simulink model "UART_test"  (R2020a)
settings: Solver=FixedStepAuto  StartTime=0.0  StopTime=10.0  FixedStep=1e-3  RelTol=1e-3  EnableMultiTasking=on
libraries: etargetslib x17, frdmk64flib x10, simulink x1
(part 2 of 3)

== stateflow chart UART_test/Pacing Modes ==
  state Pacing_Off
    % do nothing
  state Pacing_Modes_Switch
    % switch pacing modes according to MODE
    % This is similar to switch case structure in C plus plus
    % this block is executed only after mode is switched or pparams are updated
    entry:
    % Reset LEDs
    R_LED=false;
    G_LED=false;
    B_LED=false;
    % reset output variables before switching mode
    VENT_CMP_REF_PWM=100;
    ATR_CMP_REF_PWM=100;
    FRONTEND_CTRL=true;
    ATR_PACE_CTRL = false;
    VENT_PACE_CTRL = false;
    PACING_REF_PWM = 0;
    PACE_CHARGE_CTRL = false;
    PACE_GND_CTRL = false;
    Z_ATR_CTRL = false;
    Z_VENT_CTRL = false;
    ATR_GND_CTRL = false;
    VENT_GND_CTRL = false;
    % Update internal double representations of input parameters
    % Note: MODE and ACT_THRESHOLD don't need to be double
    % MODE=double(MODE_i);
    LRL=double(LRL_i);
    URL=double(URL_i);
    MAX_SENSOR_RATE=double(MAX_SENSOR_RATE_i);
    AV_DELAY_FIXED=double(AV_DELAY_FIXED_i);
    AV_DELAY_DYNAMIC=double(AV_DELAY_DYNAMIC_i);
    MIN_AV_DELAY_DYNAMIC=double(MIN_AV_DELAY_DYNAMIC_i);
    AV_DELAY_OFFSET_SENSED=double(AV_DELAY_OFFSET_SENSED_i);
    ATR_AMP_REG=double(ATR_AMP_REG_i);
    VENT_AMP_REG=double(VENT_AMP_REG_i);
    ATR_AMP_UNREG=double(ATR_AMP_UNREG_i);
    VENT_AMP_UNREG=double(VENT_AMP_UNREG_i);
    ATR_PULSE_WIDTH=double(ATR_PULSE_WIDTH_i);
    VENT_PULSE_WIDTH=double(VENT_PULSE_WIDTH_i);
    ATR_SENSITIVITY=double(ATR_SENSITIVITY_i);
    VENT_SENSITIVITY=double(VENT_SENSITIVITY_i);
    VRP=double(VRP_i);
    ARP=double(ARP_i);
    PVARP=double(PVARP_i);
    PVARP_EXT=double(PVARP_EXT_i);
    HYSTERESIS_LIMIT=double(HYSTERESIS_LIMIT_i);
    RATE_SMOOTHING=double(RATE_SMOOTHING_i);
    ATR_MODE=double(ATR_MODE_i);
    ATR_DURATION=double(ATR_DURATION_i);
    ATR_FALLBACK_TIME=double(ATR_FALLBACK_TIME_i);
    VENT_BLANKING=double(VENT_BLANKING_i);
    % ACT_THRESHOLD=double(ACT_THRESHOLD_i);
    REACTION_TIME=double(REACTION_TIME_i);
    RESPONSE_FACTOR=double(RESPONSE_FACTOR_i);
    RECOVERY_TIME=double(RECOVERY_TIME_i);
  state DOO
    note: DOO Pacing Mode:
        | equivalent to AOO combined with VOO, but with a AV_Delay
    state Atrium_Pacing
      entry:
      % VENT_PACE_CTRL = false;
      % ATR_GND_CTRL = false;
      VENT_GND_CTRL = false;
      PACE_CHARGE_CTRL = false;
      % starting pacing at last step to be secure
      ATR_PACE_CTRL = true;
    state Atrium_Charging
      %% Charge C22
      entry:
      % ATR_PACE_CTRL = false;
      VENT_PACE_CTRL = false;
      ATR_GND_CTRL = false;
      %% discharge residual voltage inside ventricle
      VENT_GND_CTRL = true;
      % Because 0-100% PWM corresponds to 0-5V output,
      % PWM duty cycle = ATR_AMP_REG/5*100;
      PACING_REF_PWM = ATR_AMP_REG*20;
      PACE_CHARGE_CTRL = true;
    state Init
      % Initialize
      entry:
      %% C21 is always connected
      PACE_GND_CTRL = true;
      Z_ATR_CTRL = false;
      Z_VENT_CTRL = false;
    state Ventricle_Pacing
      entry:
      % ATR_PACE_CTRL = false;
      ATR_GND_CTRL = false;
      % VENT_GND_CTRL = false;
      PACE_CHARGE_CTRL = false;
      % starting pacing at last step to be secure
      VENT_PACE_CTRL = true;
    state Ventricle_Charging
      % charge C22
      entry:
      ATR_PACE_CTRL = false;
      % VENT_PACE_CTRL = false;
      %% discharge residual voltage inside atrium
      ATR_GND_CTRL = true;
      VENT_GND_CTRL = false;
      % Because 0-100% PWM corresponds to 0-5V output,
      %PWM duty cycle = VENT_AMP_REG/5*100;
      PACING_REF_PWM = VENT_AMP_REG*20;
      PACE_CHARGE_CTRL = true;
    (default) -> DOO.Init
    DOO.Atrium_Charging -> DOO.Atrium_Pacing : [after(60000/LRL-ATR_PULSE_WIDTH-AV_DELAY_FIXED-VENT_PULSE_WIDTH,msec)]
    DOO.Init -> DOO.Atrium_Charging
    DOO.Atrium_Pacing -> DOO.Ventricle_Charging : [after(ATR_PULSE_WIDTH,msec)]
    DOO.Ventricle_Pacing -> DOO.Atrium_Charging : [after(VENT_PULSE_WIDTH,msec)]
    DOO.Ventricle_Charging -> DOO.Ventricle_Pacing : [after(AV_DELAY_FIXED,msec)]
  state AOO
    note: AOO Pacing Mode:
        |
        | Inputs:
        | ppm=LRL; (1/automatic interval)
        | ATR_AMP_REG; (amplitude in V)
        | ATR_PULSE_WIDTH; (in msec)
    state Charging
      %% Charge C22
      entry:
      ATR_PACE_CTRL = false;
      ATR_GND_CTRL = true;
      % Because 0-100% PWM corresponds to 0-5V output,
      % PWM duty cycle = ATR_AMP_REG/5*100;
      PACING_REF_PWM = ATR_AMP_REG*20;
      PACE_CHARGE_CTRL = true;
    state Pacing
      entry:
      ATR_GND_CTRL = false;
      PACE_CHARGE_CTRL = false;
      % start pacing at last step to be secure
      ATR_PACE_CTRL = true;
    state Init
      % Initialize
      entry:
      %% C21 is always connected
      PACE_GND_CTRL = true;
      Z_ATR_CTRL = false;
      Z_VENT_CTRL = false;
      VENT_GND_CTRL = false;
      VENT_PACE_CTRL = false;
    (default) -> AOO.Init
    AOO.Charging -> AOO.Pacing : [after(60000/LRL-ATR_PULSE_WIDTH,msec)]
    AOO.Init -> AOO.Charging
    AOO.Pacing -> AOO.Charging : [after(ATR_PULSE_WIDTH,msec)]
  state DOOR
    state Very_High_Threshold
      entry:
      % assign predefined constant
      ACT_THRESHOLD=ACT_V_HIGH;
    state High_Threshold
      entry:
      ACT_THRESHOLD=ACT_HIGH;
    state Init
      entry:
      % initialize constants that will be used in the ..._Cycle
      BPM = LRL;
      % MSR_ALTERED: max sensor rate altered to be smaller than either limit (MSR or URL)
      MSR_ALTERED=min(MAX_SENSOR_RATE,URL);
      % difference between MSR and LRL
      DIFF_MSR_LRL=MSR_ALTERED-LRL;
      % target and slope for BPM when activity higher/lower than threshold
      TARGET_HIGH = DIFF_MSR_LRL * (RESPONSE_FACTOR/16) + LRL;
      TARGET_LOW = LRL;
      SLOPE_UP=DIFF_MSR_LRL/REACTION_TIME;
      SLOPE_DOWN=DIFF_MSR_LRL/RECOVERY_TIME;
      % Note: both reaction and recovery time are in seconds
    state Medium_High_Threshold
      entry:
      ACT_THRESHOLD=ACT_M_HIGH;
    state DOOR_Cycle
      state BPM_Update [parallel]
        settings: executionOrder=1
        state Get_activity
          entry:
          ACTIVITY_NORM = sqrt(ACTIVITY(1)^2+ACTIVITY(2)^2+ACTIVITY(3)^2);
        state More_than_threshold
        state Less_than_threshold
        state Increse_HR
          entry:
          % step is change in BPM after every pace
          % the last step should be smaller to let BPM reach TARGET exactly
          STEP=min(SLOPE_UP*(60/BPM),TARGET_HIGH-BPM);
          BPM = BPM + STEP;
          B_LED=true;
          R_LED=false;
          G_LED=false;
        state Decrese_HR
          entry:
          % step is change in BPM after every pace
          % the last step should be smaller to let BPM reach TARGET exactly
          STEP=min(SLOPE_DOWN*(60/BPM),BPM-TARGET_LOW);
          BPM = BPM - STEP;
          G_LED=true;
          R_LED=false;
          B_LED=false;
        state Maintain_HR
          % no change to BPM
          entry:
          R_LED=true;
          G_LED=false;
          B_LED=false;
        (default) -> DOOR.DOOR_Cycle.BPM_Update.Get_activity
        (junction 1173) -> DOOR.DOOR_Cycle.BPM_Update.Get_activity : [after(60/BPM,sec)]
        DOOR.DOOR_Cycle.BPM_Update.Get_activity -> DOOR.DOOR_Cycle.BPM_Update.More_than_threshold [order 2] : [ACTIVITY_NORM >= ACT_THRESHOLD]
        DOOR.DOOR_Cycle.BPM_Update.Get_activity -> DOOR.DOOR_Cycle.BPM_Update.Less_than_threshold [order 1] : [ACTIVITY_NORM< ACT_THRESHOLD]
        DOOR.DOOR_Cycle.BPM_Update.Less_than_threshold -> DOOR.DOOR_Cycle.BPM_Update.Maintain_HR [order 2]
        DOOR.DOOR_Cycle.BPM_Update.Less_than_threshold -> DOOR.DOOR_Cycle.BPM_Update.Decrese_HR [order 1] : [BPM > TARGET_LOW]
        DOOR.DOOR_Cycle.BPM_Update.More_than_threshold -> DOOR.DOOR_Cycle.BPM_Update.Increse_HR [order 1] : [BPM < TARGET_HIGH]
        DOOR.DOOR_Cycle.BPM_Update.More_than_threshold -> DOOR.DOOR_Cycle.BPM_Update.Maintain_HR [order 2]
        DOOR.DOOR_Cycle.BPM_Update.Increse_HR -> (junction 1173)
        DOOR.DOOR_Cycle.BPM_Update.Maintain_HR -> (junction 1173)
        DOOR.DOOR_Cycle.BPM_Update.Decrese_HR -> (junction 1173)
      state DOO_Timing_Logic [parallel]
        settings: executionOrder=2
        note: DOO Pacing Mode:
            | equivalent to AOO combined with VOO, but with a AV_Delay
        state Atrium_Pacing
          entry:
          % VENT_PACE_CTRL = false;
          % ATR_GND_CTRL = false;
          VENT_GND_CTRL = false;
          PACE_CHARGE_CTRL = false;
          % starting pacing at last step to be secure
          ATR_PACE_CTRL = true;
        state Atrium_Charging
          %% Charge C22
          entry:
          % ATR_PACE_CTRL = false;
          VENT_PACE_CTRL = false;
          ATR_GND_CTRL = false;
          %% discharge residual voltage inside ventricle
          VENT_GND_CTRL = true;
          % Because 0-100% PWM corresponds to 0-5V output,
          % PWM duty cycle = ATR_AMP_REG/5*100;
          PACING_REF_PWM = ATR_AMP_REG*20;
          PACE_CHARGE_CTRL = true;
        state Init
          % Initialize
          entry:
          %% C21 is always connected
          PACE_GND_CTRL = true;
          Z_ATR_CTRL = false;
          Z_VENT_CTRL = false;
        state Ventricle_Pacing
          entry:
          % ATR_PACE_CTRL = false;
          ATR_GND_CTRL = false;
          % VENT_GND_CTRL = false;
          PACE_CHARGE_CTRL = false;
          % starting pacing at last step to be secure
          VENT_PACE_CTRL = true;
        state Ventricle_Charging
          % charge C22
          entry:
          ATR_PACE_CTRL = false;
          % VENT_PACE_CTRL = false;
          %% discharge residual voltage inside atrium
          ATR_GND_CTRL = true;
          VENT_GND_CTRL = false;
          % Because 0-100% PWM corresponds to 0-5V output,
          %PWM duty cycle = VENT_AMP_REG/5*100;
          PACING_REF_PWM = VENT_AMP_REG*20;
          PACE_CHARGE_CTRL = true;
        (default) -> DOOR.DOOR_Cycle.DOO_Timing_Logic.Init
        DOOR.DOOR_Cycle.DOO_Timing_Logic.Atrium_Charging -> DOOR.DOOR_Cycle.DOO_Timing_Logic.Atrium_Pacing : [after(60000/BPM - ATR_PULSE_WIDTH - AV_DELAY_FIXED - VENT_PULSE_WIDTH,msec)]
        DOOR.DOOR_Cycle.DOO_Timing_Logic.Init -> DOOR.DOOR_Cycle.DOO_Timing_Logic.Atrium_Charging
        DOOR.DOOR_Cycle.DOO_Timing_Logic.Atrium_Pacing -> DOOR.DOOR_Cycle.DOO_Timing_Logic.Ventricle_Charging : [after(ATR_PULSE_WIDTH,msec)]
        DOOR.DOOR_Cycle.DOO_Timing_Logic.Ventricle_Pacing -> DOOR.DOOR_Cycle.DOO_Timing_Logic.Atrium_Charging : [after(VENT_PULSE_WIDTH,msec)]
        DOOR.DOOR_Cycle.DOO_Timing_Logic.Ventricle_Charging -> DOOR.DOOR_Cycle.DOO_Timing_Logic.Ventricle_Pacing : [after(AV_DELAY_FIXED,msec)]
    state Medium_Threshold
      % if no match value for ACT_THRESHOLD, use medium as default
      entry:
      ACT_THRESHOLD=ACT_M;
    state Medium_Low_Threshold
      entry:
      ACT_THRESHOLD=ACT_M_LOW;
    state Low_Threshold
      entry:
      ACT_THRESHOLD=ACT_LOW;
    state Very_Low_Threshold
      entry:
      ACT_THRESHOLD=ACT_V_LOW;
    (default) -> DOOR.Init
    DOOR.Very_High_Threshold -> DOOR_Cycle
    (junction 1150) -> DOOR.Very_High_Threshold [order 1] : [ACT_THRESHOLD_i==6]
    (junction 1150) -> DOOR.High_Threshold [order 2] : [ACT_THRESHOLD_i==5]
    DOOR.High_Threshold -> DOOR_Cycle
    DOOR.Medium_High_Threshold -> DOOR_Cycle
    (junction 1150) -> DOOR.Medium_High_Threshold [order 5] : [ACT_THRESHOLD_i==4]
    DOOR.Init -> (junction 1150)
    (junction 1150) -> DOOR.Medium_Threshold [order 7]
    DOOR.Medium_Threshold -> DOOR_Cycle
    (junction 1150) -> DOOR.Medium_Low_Threshold [order 4] : [ACT_THRESHOLD_i==2]
    (junction 1150) -> DOOR.Low_Threshold [order 3] : [ACT_THRESHOLD_i==1]
    (junction 1150) -> DOOR.Very_Low_Threshold [order 6] : [ACT_THRESHOLD_i==0]
    DOOR.Low_Threshold -> DOOR_Cycle
    DOOR.Medium_Low_Threshold -> DOOR_Cycle
    DOOR.Very_Low_Threshold -> DOOR_Cycle
  state AOOR
    state Very_High_Threshold
      entry:
      % assign predefined constant
      ACT_THRESHOLD=ACT_V_HIGH;
    state High_Threshold
      entry:
      ACT_THRESHOLD=ACT_HIGH;
    state Init
      entry:
      % initialize constants that will be used in the ..._Cycle
      BPM = LRL;
      % MSR_ALTERED: max sensor rate altered to be smaller than either limit (MSR or URL)
      MSR_ALTERED=min(MAX_SENSOR_RATE,URL);
      % difference between MSR and LRL
      DIFF_MSR_LRL=MSR_ALTERED-LRL;
      % target and slope for BPM when activity higher/lower than threshold
      TARGET_HIGH = DIFF_MSR_LRL * (RESPONSE_FACTOR/16) + LRL;
      TARGET_LOW = LRL;
      SLOPE_UP=DIFF_MSR_LRL/REACTION_TIME;
      SLOPE_DOWN=DIFF_MSR_LRL/RECOVERY_TIME;
      % Note: both reaction and recovery time are in seconds
    state Medium_High_Threshold
      entry:
      ACT_THRESHOLD=ACT_M_HIGH;
    state AOOR_Cycle
      state BPM_Update [parallel]
        settings: executionOrder=1
        state Get_activity
          entry:
          ACTIVITY_NORM = sqrt(ACTIVITY(1)^2+ACTIVITY(2)^2+ACTIVITY(3)^2);
        state More_than_threshold
        state Less_than_threshold
        state Increse_HR
          entry:
          % step is change in BPM after every pace
          % the last step should be smaller to let BPM reach TARGET exactly
          STEP=min(SLOPE_UP*(60/BPM),TARGET_HIGH-BPM);
          BPM = BPM + STEP;
          B_LED=true;
          R_LED=false;
          G_LED=false;
        state Decrese_HR
          entry:
          % step is change in BPM after every pace
          % the last step should be smaller to let BPM reach TARGET exactly
          STEP=min(SLOPE_DOWN*(60/BPM),BPM-TARGET_LOW);
          BPM = BPM - STEP;
          G_LED=true;
          R_LED=false;
          B_LED=false;
        state Maintain_HR
          % no change to BPM
          entry:
          R_LED=true;
          G_LED=false;
          B_LED=false;
        (default) -> AOOR.AOOR_Cycle.BPM_Update.Get_activity
        (junction 803) -> AOOR.AOOR_Cycle.BPM_Update.Get_activity : [after(60/BPM,sec)]
        AOOR.AOOR_Cycle.BPM_Update.Get_activity -> AOOR.AOOR_Cycle.BPM_Update.More_than_threshold [order 2] : [ACTIVITY_NORM >= ACT_THRESHOLD]
        AOOR.AOOR_Cycle.BPM_Update.Get_activity -> AOOR.AOOR_Cycle.BPM_Update.Less_than_threshold [order 1] : [ACTIVITY_NORM< ACT_THRESHOLD]
        AOOR.AOOR_Cycle.BPM_Update.Less_than_threshold -> AOOR.AOOR_Cycle.BPM_Update.Maintain_HR [order 2]
        AOOR.AOOR_Cycle.BPM_Update.Less_than_threshold -> AOOR.AOOR_Cycle.BPM_Update.Decrese_HR [order 1] : [BPM > TARGET_LOW]
        AOOR.AOOR_Cycle.BPM_Update.More_than_threshold -> AOOR.AOOR_Cycle.BPM_Update.Increse_HR [order 1] : [BPM < TARGET_HIGH]
        AOOR.AOOR_Cycle.BPM_Update.More_than_threshold -> AOOR.AOOR_Cycle.BPM_Update.Maintain_HR [order 2]
        AOOR.AOOR_Cycle.BPM_Update.Increse_HR -> (junction 803)
        AOOR.AOOR_Cycle.BPM_Update.Maintain_HR -> (junction 803)
        AOOR.AOOR_Cycle.BPM_Update.Decrese_HR -> (junction 803)
      state AOO_Timing_Logic [parallel]
        settings: executionOrder=2
        note: AOO Pacing Mode:
            |
            | Inputs:
            | ppm=LRL; (1/automatic interval)
            | ATR_AMP_REG; (amplitude in V)
            | ATR_PULSE_WIDTH; (in msec)
        state Charging
          %% Charge C22
          entry:
          ATR_PACE_CTRL = false;
          ATR_GND_CTRL = true;
          % Because 0-100% PWM corresponds to 0-5V output,
          % PWM duty cycle = ATR_AMP_REG/5*100;
          PACING_REF_PWM = ATR_AMP_REG*20;
          PACE_CHARGE_CTRL = true;
        state Pacing
          entry:
          ATR_GND_CTRL = false;
          PACE_CHARGE_CTRL = false;
          ATR_PACE_CTRL = true;
        state Init
          % Initialize
          entry:
          %% C21 is always connected
          PACE_GND_CTRL = true;
          Z_ATR_CTRL = false;
          Z_VENT_CTRL = false;
          VENT_GND_CTRL = false;
          VENT_PACE_CTRL = false;
        (default) -> AOOR.AOOR_Cycle.AOO_Timing_Logic.Init
        AOOR.AOOR_Cycle.AOO_Timing_Logic.Charging -> AOOR.AOOR_Cycle.AOO_Timing_Logic.Pacing : [after(60000/BPM-ATR_PULSE_WIDTH,msec)]
        AOOR.AOOR_Cycle.AOO_Timing_Logic.Init -> AOOR.AOOR_Cycle.AOO_Timing_Logic.Charging
        AOOR.AOOR_Cycle.AOO_Timing_Logic.Pacing -> AOOR.AOOR_Cycle.AOO_Timing_Logic.Charging : [after(ATR_PULSE_WIDTH,msec)]
    state Medium_Threshold
      % if no match value for ACT_THRESHOLD, use medium as default
      entry:
      ACT_THRESHOLD=ACT_M;
    state Medium_Low_Threshold
      entry:
      ACT_THRESHOLD=ACT_M_LOW;
    state Low_Threshold
      entry:
      ACT_THRESHOLD=ACT_LOW;
    state Very_Low_Threshold
      entry:
      ACT_THRESHOLD=ACT_V_LOW;
    (default) -> AOOR.Init
    AOOR.Very_High_Threshold -> AOOR_Cycle
    (junction 148) -> AOOR.Very_High_Threshold [order 1] : [ACT_THRESHOLD_i==6]
    (junction 148) -> AOOR.High_Threshold [order 2] : [ACT_THRESHOLD_i==5]
    AOOR.High_Threshold -> AOOR_Cycle
    AOOR.Medium_High_Threshold -> AOOR_Cycle
    (junction 148) -> AOOR.Medium_High_Threshold [order 5] : [ACT_THRESHOLD_i==4]
    AOOR.Init -> (junction 148)
    (junction 148) -> AOOR.Medium_Threshold [order 7]
    AOOR.Medium_Threshold -> AOOR_Cycle
    (junction 148) -> AOOR.Medium_Low_Threshold [order 4] : [ACT_THRESHOLD_i==2]
    (junction 148) -> AOOR.Low_Threshold [order 3] : [ACT_THRESHOLD_i==1]
    (junction 148) -> AOOR.Very_Low_Threshold [order 6] : [ACT_THRESHOLD_i==0]
    AOOR.Low_Threshold -> AOOR_Cycle
    AOOR.Medium_Low_Threshold -> AOOR_Cycle
    AOOR.Very_Low_Threshold -> AOOR_Cycle
  state VOO
    note: VOO Pacing Mode:
        |
        | Inputs:
        | ppm=LRL; (1/automatic interval)
        | VENT_AMP_REG; (amplitude in V)
        | VENT_PULSE_WIDTH; (in msec)
    state Charging1
      %% Charge C22
      entry:
      VENT_PACE_CTRL = false;
      VENT_GND_CTRL = true;
      % Because 0-100% PWM corresponds to 0-5V output,
      % PWM duty cycle = VENT_AMP_REG/5*100;
      PACING_REF_PWM = VENT_AMP_REG*20;
      PACE_CHARGE_CTRL = true;
    state Pacing1
      entry:
      VENT_GND_CTRL = false;
      PACE_CHARGE_CTRL = false;
      % start pacing at last step to be secure
      VENT_PACE_CTRL = true;
    state Init
      % Initialize
      entry:
      %% C21 is always connected
      PACE_GND_CTRL = true;
      Z_ATR_CTRL = false;
      Z_VENT_CTRL = false;
      ATR_GND_CTRL = false;
      ATR_PACE_CTRL = false;
    (default) -> VOO.Init
    VOO.Charging1 -> VOO.Pacing1 : [after(60000/LRL-VENT_PULSE_WIDTH,msec)]
    VOO.Init -> VOO.Charging1
    VOO.Pacing1 -> VOO.Charging1 : [after(VENT_PULSE_WIDTH,msec)]
  state VOOR
    state Very_High_Threshold
      entry:
      % assign predefined constant
      ACT_THRESHOLD=ACT_V_HIGH;
    state High_Threshold
      entry:
      ACT_THRESHOLD=ACT_HIGH;
    state Init
      entry:
      % initialize constants that will be used in the ..._Cycle
      BPM = LRL;
      % MSR_ALTERED: max sensor rate altered to be smaller than either limit (MSR or URL)
      MSR_ALTERED=min(MAX_SENSOR_RATE,URL);
      % difference between MSR and LRL
      DIFF_MSR_LRL=MSR_ALTERED-LRL;
      % target and slope for BPM when activity higher/lower than threshold
      TARGET_HIGH = DIFF_MSR_LRL * (RESPONSE_FACTOR/16) + LRL;
      TARGET_LOW = LRL;
      SLOPE_UP=DIFF_MSR_LRL/REACTION_TIME;
      SLOPE_DOWN=DIFF_MSR_LRL/RECOVERY_TIME;
      % Note: both reaction and recovery time are in seconds
    state Medium_High_Threshold
      entry:
      ACT_THRESHOLD=ACT_M_HIGH;
    state VOOR_Cycle
      state BPM_Update [parallel]
        settings: executionOrder=1
        state Get_activity
          entry:
          ACTIVITY_NORM = sqrt(ACTIVITY(1)^2+ACTIVITY(2)^2+ACTIVITY(3)^2);
        state More_than_threshold
        state Less_than_threshold
        state Increse_HR
          entry:
          % step is change in BPM after every pace
          % the last step should be smaller to let BPM reach TARGET exactly
          STEP=min(SLOPE_UP*(60/BPM),TARGET_HIGH-BPM);
          BPM = BPM + STEP;
          B_LED=true;
          R_LED=false;
          G_LED=false;
        state Decrese_HR
          entry:
          % step is change in BPM after every pace
          % the last step should be smaller to let BPM reach TARGET exactly
          STEP=min(SLOPE_DOWN*(60/BPM),BPM-TARGET_LOW);
          BPM = BPM - STEP;
          G_LED=true;
          R_LED=false;
          B_LED=false;
        state Maintain_HR
          % no change to BPM
          entry:
          R_LED=true;
          G_LED=false;
          B_LED=false;
        (default) -> VOOR.VOOR_Cycle.BPM_Update.Get_activity
        (junction 972) -> VOOR.VOOR_Cycle.BPM_Update.Get_activity : [after(60/BPM,sec)]
        VOOR.VOOR_Cycle.BPM_Update.Get_activity -> VOOR.VOOR_Cycle.BPM_Update.More_than_threshold [order 2] : [ACTIVITY_NORM >= ACT_THRESHOLD]
        VOOR.VOOR_Cycle.BPM_Update.Get_activity -> VOOR.VOOR_Cycle.BPM_Update.Less_than_threshold [order 1] : [ACTIVITY_NORM< ACT_THRESHOLD]
        VOOR.VOOR_Cycle.BPM_Update.Less_than_threshold -> VOOR.VOOR_Cycle.BPM_Update.Maintain_HR [order 2]
        VOOR.VOOR_Cycle.BPM_Update.Less_than_threshold -> VOOR.VOOR_Cycle.BPM_Update.Decrese_HR [order 1] : [BPM > TARGET_LOW]
        VOOR.VOOR_Cycle.BPM_Update.More_than_threshold -> VOOR.VOOR_Cycle.BPM_Update.Increse_HR [order 1] : [BPM < TARGET_HIGH]
        VOOR.VOOR_Cycle.BPM_Update.More_than_threshold -> VOOR.VOOR_Cycle.BPM_Update.Maintain_HR [order 2]
        VOOR.VOOR_Cycle.BPM_Update.Increse_HR -> (junction 972)
        VOOR.VOOR_Cycle.BPM_Update.Maintain_HR -> (junction 972)
        VOOR.VOOR_Cycle.BPM_Update.Decrese_HR -> (junction 972)
      state VOO_Timing_Logic [parallel]
        settings: executionOrder=2
        note: VOO Pacing Mode:
            |
            | Inputs:
            | ppm=LRL; (1/automatic interval)
            | VENT_AMP_REG; (amplitude in V)
            | VENT_PULSE_WIDTH; (in msec)
        state Charging1
          %% Charge C22
          entry:
          VENT_PACE_CTRL = false;
          VENT_GND_CTRL = true;
          % Because 0-100% PWM corresponds to 0-5V output,
          % PWM duty cycle = VENT_AMP_REG/5*100;
          PACING_REF_PWM = VENT_AMP_REG*20;
          PACE_CHARGE_CTRL = true;
        state Pacing1
          entry:
          VENT_GND_CTRL = false;
          PACE_CHARGE_CTRL = false;
          % start pacing at last step to be secure
          VENT_PACE_CTRL = true;
        state Init
          % Initialize
          entry:
          %% C21 is always connected
          PACE_GND_CTRL = true;
          Z_ATR_CTRL = false;
          Z_VENT_CTRL = false;
          ATR_GND_CTRL = false;
          ATR_PACE_CTRL = false;
        (default) -> VOOR.VOOR_Cycle.VOO_Timing_Logic.Init
        VOOR.VOOR_Cycle.VOO_Timing_Logic.Charging1 -> VOOR.VOOR_Cycle.VOO_Timing_Logic.Pacing1 : [after(60000/BPM-VENT_PULSE_WIDTH,msec)]
        VOOR.VOOR_Cycle.VOO_Timing_Logic.Init -> VOOR.VOOR_Cycle.VOO_Timing_Logic.Charging1
        VOOR.VOOR_Cycle.VOO_Timing_Logic.Pacing1 -> VOOR.VOOR_Cycle.VOO_Timing_Logic.Charging1 : [after(VENT_PULSE_WIDTH,msec)]
    state Medium_Threshold
      % if no match value for ACT_THRESHOLD, use medium as default
      entry:
      ACT_THRESHOLD=ACT_M;
    state Medium_Low_Threshold
      entry:
      ACT_THRESHOLD=ACT_M_LOW;
    state Low_Threshold
      entry:
      ACT_THRESHOLD=ACT_LOW;
    state Very_Low_Threshold
      entry:
      ACT_THRESHOLD=ACT_V_LOW;
    (default) -> VOOR.Init
    VOOR.Very_High_Threshold -> VOOR_Cycle
    (junction 949) -> VOOR.Very_High_Threshold [order 1] : [ACT_THRESHOLD_i==6]
    (junction 949) -> VOOR.High_Threshold [order 2] : [ACT_THRESHOLD_i==5]
    VOOR.High_Threshold -> VOOR_Cycle
    VOOR.Medium_High_Threshold -> VOOR_Cycle
    (junction 949) -> VOOR.Medium_High_Threshold [order 5] : [ACT_THRESHOLD_i==4]
    VOOR.Init -> (junction 949)
    (junction 949) -> VOOR.Medium_Threshold [order 7]
    VOOR.Medium_Threshold -> VOOR_Cycle
    (junction 949) -> VOOR.Medium_Low_Threshold [order 4] : [ACT_THRESHOLD_i==2]
    (junction 949) -> VOOR.Low_Threshold [order 3] : [ACT_THRESHOLD_i==1]
    (junction 949) -> VOOR.Very_Low_Threshold [order 6] : [ACT_THRESHOLD_i==0]
    VOOR.Low_Threshold -> VOOR_Cycle
    VOOR.Medium_Low_Threshold -> VOOR_Cycle
    VOOR.Very_Low_Threshold -> VOOR_Cycle
  state AAI
    state REF_delay
    note: AAI Pacing Mode:
        | Inputs:
        | ATR_SENSITIVITY (sensing threshold in V)
        | ARP; (atrial refactory period, in msec)
        | ppm= LRL; (1/automatic interval)
        | ATR_AMP_REG (amplitude in V)
        | ATR_PULSE_WIDTH; (pulse width in msec)
        | ATR_CMP_DETECT; (sensing signal from hardware)
    state Init_Sensing
      entry:
      % see explanation for ...REF_PWM in section 2.3.4 of the Document
      ATR_CMP_REF_PWM = ATR_SENSITIVITY*20;
      %% C21 is always connected
      PACE_GND_CTRL = true;
      Z_ATR_CTRL = false;
      Z_VENT_CTRL = false;
      VENT_GND_CTRL = false;
      VENT_PACE_CTRL = false;
    state Charging1
      %% Charge C22
      entry:
      ATR_PACE_CTRL = false;
      ATR_GND_CTRL = true;
      % Because 0-100% PWM corresponds to 0-5V output,
      % PWM duty cycle = ATR_AMP_REG/5*100;
      PACING_REF_PWM = ATR_AMP_REG*20;
      PACE_CHARGE_CTRL = true;
    state Pacing
      entry:
      ATR_GND_CTRL = false;
      PACE_CHARGE_CTRL = false;
      % start pacing at last step to be secure
      ATR_PACE_CTRL = true;
    AAI.REF_delay -> AAI.Pacing [order 1] : [after(60000/LRL - ATR_PULSE_WIDTH - ARP, msec)]
    AAI.Charging1 -> AAI.REF_delay : [after(ARP,msec)]
    AAI.REF_delay -> AAI.Charging1 [order 2] : [ATR_CMP_DETECT == true || PUSH_BUTTON==true]
    (default) -> AAI.Init_Sensing
    AAI.Init_Sensing -> AAI.Charging1
    AAI.Pacing -> AAI.Charging1 : [after(ATR_PULSE_WIDTH,msec)]
  state AAIR
    state Very_High_Threshold
      entry:
      % assign predefined constant
      ACT_THRESHOLD=ACT_V_HIGH;
    state High_Threshold
      entry:
      ACT_THRESHOLD=ACT_HIGH;
    state Init
      entry:
      % initialize constants that will be used in the ..._Cycle
      BPM = LRL;
      % MSR_ALTERED: max sensor rate altered to be smaller than either limit (MSR or URL)
      MSR_ALTERED=min(MAX_SENSOR_RATE,URL);
      % difference between MSR and LRL
      DIFF_MSR_LRL=MSR_ALTERED-LRL;
      % target and slope for BPM when activity higher/lower than threshold
      TARGET_HIGH = DIFF_MSR_LRL * (RESPONSE_FACTOR/16) + LRL;
      TARGET_LOW = LRL;
      SLOPE_UP=DIFF_MSR_LRL/REACTION_TIME;
      SLOPE_DOWN=DIFF_MSR_LRL/RECOVERY_TIME;
      % Note: both reaction and recovery time are in seconds
    state Medium_High_Threshold
      entry:
      ACT_THRESHOLD=ACT_M_HIGH;
    state AAIR_Cycle
      state BPM_Update [parallel]
        settings: executionOrder=1
        state Get_activity
          entry:
          ACTIVITY_NORM = sqrt(ACTIVITY(1)^2+ACTIVITY(2)^2+ACTIVITY(3)^2);
        state More_than_threshold
        state Less_than_threshold
        state Increse_HR
          entry:
          % step is change in BPM after every pace
          % the last step should be smaller to let BPM reach TARGET exactly
          STEP=min(SLOPE_UP*(60/BPM),TARGET_HIGH-BPM);
          BPM = BPM + STEP;
          B_LED=true;
          R_LED=false;
          G_LED=false;
        state Decrese_HR
          entry:
          % step is change in BPM after every pace
          % the last step should be smaller to let BPM reach TARGET exactly
          STEP=min(SLOPE_DOWN*(60/BPM),BPM-TARGET_LOW);
          BPM = BPM - STEP;
          G_LED=true;
          R_LED=false;
          B_LED=false;
        state Maintain_HR
          % no change to BPM
          entry:
          R_LED=true;
          G_LED=false;
          B_LED=false;
        (default) -> AAIR.AAIR_Cycle.BPM_Update.Get_activity
        (junction 1024) -> AAIR.AAIR_Cycle.BPM_Update.Get_activity : [after(60/BPM,sec)]
        AAIR.AAIR_Cycle.BPM_Update.Get_activity -> AAIR.AAIR_Cycle.BPM_Update.More_than_threshold [order 2] : [ACTIVITY_NORM >= ACT_THRESHOLD]
        AAIR.AAIR_Cycle.BPM_Update.Get_activity -> AAIR.AAIR_Cycle.BPM_Update.Less_than_threshold [order 1] : [ACTIVITY_NORM< ACT_THRESHOLD]
        AAIR.AAIR_Cycle.BPM_Update.Less_than_threshold -> AAIR.AAIR_Cycle.BPM_Update.Maintain_HR [order 2]
        AAIR.AAIR_Cycle.BPM_Update.Less_than_threshold -> AAIR.AAIR_Cycle.BPM_Update.Decrese_HR [order 1] : [BPM > TARGET_LOW]
        AAIR.AAIR_Cycle.BPM_Update.More_than_threshold -> AAIR.AAIR_Cycle.BPM_Update.Increse_HR [order 1] : [BPM < TARGET_HIGH]
        AAIR.AAIR_Cycle.BPM_Update.More_than_threshold -> AAIR.AAIR_Cycle.BPM_Update.Maintain_HR [order 2]
        AAIR.AAIR_Cycle.BPM_Update.Increse_HR -> (junction 1024)
        AAIR.AAIR_Cycle.BPM_Update.Maintain_HR -> (junction 1024)
        AAIR.AAIR_Cycle.BPM_Update.Decrese_HR -> (junction 1024)
      state AAI_Timing_Logic [parallel]
        settings: executionOrder=2
        state REF_delay
        note: AAI Pacing Mode:
            | Inputs:
            | ATR_SENSITIVITY (sensing threshold in V)
            | ARP; (atrial refactory period, in msec)
            | ppm= LRL; (1/automatic interval)
            | ATR_AMP_REG (amplitude in V)
            | ATR_PULSE_WIDTH; (pulse width in msec)
            | ATR_CMP_DETECT; (sensing signal from hardware)
        state Init_Sensing
          entry:
          % see explanation for ...REF_PWM in section 2.3.4 of the Document
          ATR_CMP_REF_PWM = ATR_SENSITIVITY*20;
          %% C21 is always connected
          PACE_GND_CTRL = true;
          Z_ATR_CTRL = false;
          Z_VENT_CTRL = false;
          VENT_GND_CTRL = false;
          VENT_PACE_CTRL = false;
        state Charging
          %% Charge C22
          entry:
          ATR_PACE_CTRL = false;
          ATR_GND_CTRL = true;
          % Because 0-100% PWM corresponds to 0-5V output,
          % PWM duty cycle = ATR_AMP_REG/5*100;
          PACING_REF_PWM = ATR_AMP_REG*20;
          PACE_CHARGE_CTRL = true;
        state Pacing
          entry:
          ATR_GND_CTRL = false;
          PACE_CHARGE_CTRL = false;
          % start pacing at last step to be secure
          ATR_PACE_CTRL = true;
        AAIR.AAIR_Cycle.AAI_Timing_Logic.REF_delay -> AAIR.AAIR_Cycle.AAI_Timing_Logic.Pacing [order 1] : [after(60000/BPM - ATR_PULSE_WIDTH - ARP, msec)]
        AAIR.AAIR_Cycle.AAI_Timing_Logic.Charging -> AAIR.AAIR_Cycle.AAI_Timing_Logic.REF_delay : [after(ARP,msec)]
        AAIR.AAIR_Cycle.AAI_Timing_Logic.REF_delay -> AAIR.AAIR_Cycle.AAI_Timing_Logic.Charging [order 2] : [ATR_CMP_DETECT == true || PUSH_BUTTON==true]
        (default) -> AAIR.AAIR_Cycle.AAI_Timing_Logic.Init_Sensing
        AAIR.AAIR_Cycle.AAI_Timing_Logic.Init_Sensing -> AAIR.AAIR_Cycle.AAI_Timing_Logic.Charging
        AAIR.AAIR_Cycle.AAI_Timing_Logic.Pacing -> AAIR.AAIR_Cycle.AAI_Timing_Logic.Charging : [after(ATR_PULSE_WIDTH,msec)]
    state Medium_Threshold
      % if no match value for ACT_THRESHOLD, use medium as default
      entry:
      ACT_THRESHOLD=ACT_M;
    state Medium_Low_Threshold
      entry:
      ACT_THRESHOLD=ACT_M_LOW;
    state Low_Threshold
      entry:
      ACT_THRESHOLD=ACT_LOW;
    state Very_Low_Threshold
      entry:
      ACT_THRESHOLD=ACT_V_LOW;
    (default) -> AAIR.Init
    AAIR.Very_High_Threshold -> AAIR_Cycle
    (junction 1001) -> AAIR.Very_High_Threshold [order 1] : [ACT_THRESHOLD_i==6]
    (junction 1001) -> AAIR.High_Threshold [order 2] : [ACT_THRESHOLD_i==5]
    AAIR.High_Threshold -> AAIR_Cycle
    AAIR.Medium_High_Threshold -> AAIR_Cycle
    (junction 1001) -> AAIR.Medium_High_Threshold [order 5] : [ACT_THRESHOLD_i==4]
    AAIR.Init -> (junction 1001)
    (junction 1001) -> AAIR.Medium_Threshold [order 7]
    AAIR.Medium_Threshold -> AAIR_Cycle
    (junction 1001) -> AAIR.Medium_Low_Threshold [order 4] : [ACT_THRESHOLD_i==2]
    (junction 1001) -> AAIR.Low_Threshold [order 3] : [ACT_THRESHOLD_i==1]
    (junction 1001) -> AAIR.Very_Low_Threshold [order 6] : [ACT_THRESHOLD_i==0]
    AAIR.Low_Threshold -> AAIR_Cycle
    AAIR.Medium_Low_Threshold -> AAIR_Cycle
    AAIR.Very_Low_Threshold -> AAIR_Cycle
  state VVI
    note: VVI Pacing Mode:
        | Inputs
        | VENT_SENSITIVITY; (sensing threshold in V)
        | VRP; (ventricular refactory period, in msec)
        | ppm=LRL; (1/automatic interval)
        | VENT_AMP; (amplitude in V)
        | VENT_PULSE_WIDTH; (in msec)
        | VENT_CMP_DETECT (sensing signal from hardware)
    state REF_delay
    state Init_Sensing1
      entry:
      % see explanation for ...REF_PWM in section 2.3.4 of the Document
      VENT_CMP_REF_PWM =VENT_SENSITIVITY*20;
      %% C21 is always connected
      PACE_GND_CTRL = true;
      Z_ATR_CTRL = false;
      Z_VENT_CTRL = false;
      ATR_GND_CTRL = false;
      ATR_PACE_CTRL = false;
    state Charging
      %% Charge C22
      entry:
      VENT_PACE_CTRL = false;
      VENT_GND_CTRL = true;
      % Because 0-100% PWM corresponds to 0-5V output,
      % PWM duty cycle = VENT_AMP_REG/5*100;
      PACING_REF_PWM = VENT_AMP_REG*20;
      PACE_CHARGE_CTRL = true;
    state Pacing2
      entry:
      VENT_GND_CTRL = false;
      PACE_CHARGE_CTRL = false;
      % start pacing at last step to be secure
      VENT_PACE_CTRL = true;
    VVI.REF_delay -> VVI.Pacing2 [order 1] : [after(60000/LRL - VENT_PULSE_WIDTH - VRP, msec)]
    VVI.Charging -> VVI.REF_delay : [after(VRP,msec)]
    VVI.REF_delay -> VVI.Charging [order 2] : [VENT_CMP_DETECT == true || PUSH_BUTTON==true]
    (default) -> VVI.Init_Sensing1
    VVI.Init_Sensing1 -> VVI.Charging
    VVI.Pacing2 -> VVI.Charging : [after(VENT_PULSE_WIDTH,msec)]
  state VVIR
    state Very_High_Threshold
      entry:
      % assign predefined constant
      ACT_THRESHOLD=ACT_V_HIGH;
    state High_Threshold
      entry:
      ACT_THRESHOLD=ACT_HIGH;
    state Init
      entry:
      % initialize constants that will be used in the ..._Cycle
      BPM = LRL;
      % MSR_ALTERED: max sensor rate altered to be smaller than either limit (MSR or URL)
      MSR_ALTERED=min(MAX_SENSOR_RATE,URL);
      % difference between MSR and LRL
      DIFF_MSR_LRL=MSR_ALTERED-LRL;
      % target and slope for BPM when activity higher/lower than threshold
      TARGET_HIGH = DIFF_MSR_LRL * (RESPONSE_FACTOR/16) + LRL;
      TARGET_LOW = LRL;
      SLOPE_UP=DIFF_MSR_LRL/REACTION_TIME;
      SLOPE_DOWN=DIFF_MSR_LRL/RECOVERY_TIME;
      % Note: both reaction and recovery time are in seconds
    state Medium_High_Threshold
      entry:
      ACT_THRESHOLD=ACT_M_HIGH;
    state VVIR_Cycle
      state BPM_Update [parallel]
        settings: executionOrder=1
        state Get_activity
          entry:
          ACTIVITY_NORM = sqrt(ACTIVITY(1)^2+ACTIVITY(2)^2+ACTIVITY(3)^2);
        state More_than_threshold
        state Less_than_threshold
        state Increse_HR
          entry:
          % step is change in BPM after every pace
          % the last step should be smaller to let BPM reach TARGET exactly
          STEP=min(SLOPE_UP*(60/BPM),TARGET_HIGH-BPM);
          BPM = BPM + STEP;
          B_LED=true;
          R_LED=false;
          G_LED=false;
        state Decrese_HR
          entry:
          % step is change in BPM after every pace
          % the last step should be smaller to let BPM reach TARGET exactly
          STEP=min(SLOPE_DOWN*(60/BPM),BPM-TARGET_LOW);
          BPM = BPM - STEP;
          G_LED=true;
          R_LED=false;
          B_LED=false;
        state Maintain_HR
          % no change to BPM
          entry:
          R_LED=true;
          G_LED=false;
          B_LED=false;
        (default) -> VVIR.VVIR_Cycle.BPM_Update.Get_activity
        (junction 1076) -> VVIR.VVIR_Cycle.BPM_Update.Get_activity : [after(60/BPM,sec)]
        VVIR.VVIR_Cycle.BPM_Update.Get_activity -> VVIR.VVIR_Cycle.BPM_Update.More_than_threshold [order 2] : [ACTIVITY_NORM >= ACT_THRESHOLD]
        VVIR.VVIR_Cycle.BPM_Update.Get_activity -> VVIR.VVIR_Cycle.BPM_Update.Less_than_threshold [order 1] : [ACTIVITY_NORM< ACT_THRESHOLD]
        VVIR.VVIR_Cycle.BPM_Update.Less_than_threshold -> VVIR.VVIR_Cycle.BPM_Update.Maintain_HR [order 2]
        VVIR.VVIR_Cycle.BPM_Update.Less_than_threshold -> VVIR.VVIR_Cycle.BPM_Update.Decrese_HR [order 1] : [BPM > TARGET_LOW]
        VVIR.VVIR_Cycle.BPM_Update.More_than_threshold -> VVIR.VVIR_Cycle.BPM_Update.Increse_HR [order 1] : [BPM < TARGET_HIGH]
        VVIR.VVIR_Cycle.BPM_Update.More_than_threshold -> VVIR.VVIR_Cycle.BPM_Update.Maintain_HR [order 2]
        VVIR.VVIR_Cycle.BPM_Update.Increse_HR -> (junction 1076)
        VVIR.VVIR_Cycle.BPM_Update.Maintain_HR -> (junction 1076)
        VVIR.VVIR_Cycle.BPM_Update.Decrese_HR -> (junction 1076)
      state VVI_Timing_Logic [parallel]
        settings: executionOrder=2
        note: VVI Pacing Mode:
            | Inputs
            | VENT_SENSITIVITY; (sensing threshold in V)
            | VRP; (ventricular refactory period, in msec)
            | ppm=LRL; (1/automatic interval)
            | VENT_AMP; (amplitude in V)
            | VENT_PULSE_WIDTH; (in msec)
            | VENT_CMP_DETECT (sensing signal from hardware)
        state REF_delay
        state Init_Sensing1
          entry:
          % see explanation for ...REF_PWM in section 2.3.4 of the Document
          VENT_CMP_REF_PWM =VENT_SENSITIVITY*20;
          %% C21 is always connected
          PACE_GND_CTRL = true;
          Z_ATR_CTRL = false;
          Z_VENT_CTRL = false;
          ATR_GND_CTRL = false;
          ATR_PACE_CTRL = false;
        state Charging
          %% Charge C22
          entry:
          VENT_PACE_CTRL = false;
          VENT_GND_CTRL = true;
          % Because 0-100% PWM corresponds to 0-5V output,
          % PWM duty cycle = VENT_AMP_REG/5*100;
          PACING_REF_PWM = VENT_AMP_REG*20;
          PACE_CHARGE_CTRL = true;
        state Pacing2
          entry:
          VENT_GND_CTRL = false;
          PACE_CHARGE_CTRL = false;
          % start pacing at last step to be secure
          VENT_PACE_CTRL = true;
        VVIR.VVIR_Cycle.VVI_Timing_Logic.REF_delay -> VVIR.VVIR_Cycle.VVI_Timing_Logic.Pacing2 [order 1] : [after(60000/BPM - VENT_PULSE_WIDTH - VRP, msec)]
        VVIR.VVIR_Cycle.VVI_Timing_Logic.Charging -> VVIR.VVIR_Cycle.VVI_Timing_Logic.REF_delay : [after(VRP,msec)]
        VVIR.VVIR_Cycle.VVI_Timing_Logic.REF_delay -> VVIR.VVIR_Cycle.VVI_Timing_Logic.Charging [order 2] : [VENT_CMP_DETECT == true || PUSH_BUTTON==true]
        (default) -> VVIR.VVIR_Cycle.VVI_Timing_Logic.Init_Sensing1
        VVIR.VVIR_Cycle.VVI_Timing_Logic.Init_Sensing1 -> VVIR.VVIR_Cycle.VVI_Timing_Logic.Charging
        VVIR.VVIR_Cycle.VVI_Timing_Logic.Pacing2 -> VVIR.VVIR_Cycle.VVI_Timing_Logic.Charging : [after(VENT_PULSE_WIDTH,msec)]
    state Medium_Threshold
      % if no match value for ACT_THRESHOLD, use medium as default
      entry:
      ACT_THRESHOLD=ACT_M;
    state Medium_Low_Threshold
      entry:
      ACT_THRESHOLD=ACT_M_LOW;
    state Low_Threshold
      entry:
      ACT_THRESHOLD=ACT_LOW;
    state Very_Low_Threshold
      entry:
      ACT_THRESHOLD=ACT_V_LOW;
    (default) -> VVIR.Init
    VVIR.Very_High_Threshold -> VVIR_Cycle
    (junction 1053) -> VVIR.Very_High_Threshold [order 1] : [ACT_THRESHOLD_i==6]
    VVIR.High_Threshold -> VVIR_Cycle
    (junction 1053) -> VVIR.High_Threshold [order 2] : [ACT_THRESHOLD_i==5]
    VVIR.Medium_High_Threshold -> VVIR_Cycle
    (junction 1053) -> VVIR.Medium_High_Threshold [order 5] : [ACT_THRESHOLD_i==4]
    VVIR.Init -> (junction 1053)
    (junction 1053) -> VVIR.Medium_Threshold [order 7]
    VVIR.Medium_Threshold -> VVIR_Cycle
    (junction 1053) -> VVIR.Medium_Low_Threshold [order 4] : [ACT_THRESHOLD_i==2]
    (junction 1053) -> VVIR.Low_Threshold [order 3] : [ACT_THRESHOLD_i==1]
    (junction 1053) -> VVIR.Very_Low_Threshold [order 6] : [ACT_THRESHOLD_i==0]
    VVIR.Low_Threshold -> VVIR_Cycle
    VVIR.Medium_Low_Threshold -> VVIR_Cycle
    VVIR.Very_Low_Threshold -> VVIR_Cycle
  Pacing_Modes_Switch -> Pacing_Off [order 1] : [MODE==0]
  Pacing_Off -> Pacing_Modes_Switch : [MODE~=0 || PPARAM_UPDATE==true]
  (default) -> Pacing_Modes_Switch
  Pacing_Modes_Switch -> DOO [order 2] : [MODE==4]
  Pacing_Modes_Switch -> AOO [order 8] : [MODE==5]
  DOO -> Pacing_Modes_Switch : [MODE~=4 || PPARAM_UPDATE==true]
  AOO -> Pacing_Modes_Switch : [MODE~=5 || PPARAM_UPDATE==true]
  Pacing_Modes_Switch -> DOOR [order 3] : [MODE==14]
  DOOR -> Pacing_Modes_Switch : [MODE~=14 || PPARAM_UPDATE==true]
  Pacing_Modes_Switch -> AOOR [order 4] : [MODE==15]
  AOOR -> Pacing_Modes_Switch : [MODE~=15 || PPARAM_UPDATE==true]
  Pacing_Modes_Switch -> VOO [order 9] : [MODE==7]
  VOO -> Pacing_Modes_Switch : [MODE~=7 || PPARAM_UPDATE==true]
  Pacing_Modes_Switch -> VOOR [order 11] : [MODE==17]
  VOOR -> Pacing_Modes_Switch : [MODE~=17 || PPARAM_UPDATE==true]
  Pacing_Modes_Switch -> AAI [order 7] : [MODE==6]
  AAI -> Pacing_Modes_Switch : [MODE~=6 || PPARAM_UPDATE==true]
  Pacing_Modes_Switch -> AAIR [order 5] : [MODE==16]
  AAIR -> Pacing_Modes_Switch : [MODE~=16 || PPARAM_UPDATE==true]
  Pacing_Modes_Switch -> VVI [order 10] : [MODE==8]
  VVI -> Pacing_Modes_Switch : [MODE~=8 || PPARAM_UPDATE==true]
  Pacing_Modes_Switch -> VVIR [order 6] : [MODE==18]
  VVIR -> Pacing_Modes_Switch : [MODE~=18 || PPARAM_UPDATE==true]
  data: VENT_CMP_DETECT input boolean size=1; ATR_CMP_DETECT input boolean size=1; PACE_CHARGE_CTRL output boolean; VENT_CMP_REF_PWM output double; Z_ATR_CTRL output boolean; PUSH_BUTTON input boolean; PACING_REF_PWM output double; ATR_CMP_REF_PWM output double; Z_VENT_CTRL output boolean; ATR_PACE_CTRL output boolean; VENT_PACE_CTRL output boolean; PACE_GND_CTRL output boolean; ATR_GND_CTRL output boolean; VENT_GND_CTRL output boolean; FRONTEND_CTRL output boolean; MODE input uint8; LRL_i input uint8; URL_i input uint8; MAX_SENSOR_RATE_i input uint8; AV_DELAY_FIXED_i input uint16; AV_DELAY_DYNAMIC_i input uint8; MIN_AV_DELAY_DYNAMIC_i input uint8; AV_DELAY_OFFSET_SENSED_i input int8; ATR_AMP_REG_i input single; VENT_AMP_REG_i input single; ATR_AMP_UNREG_i input single; VENT_AMP_UNREG_i input single; ATR_PULSE_WIDTH_i input uint8; VENT_PULSE_WIDTH_i input uint8; ATR_SENSITIVITY_i input single; VENT_SENSITIVITY_i input single; VRP_i input uint16; ARP_i input uint16; PVARP_i input uint16; PVARP_EXT_i input uint16; HYSTERESIS_LIMIT_i input uint8; RATE_SMOOTHING_i input uint8; ATR_MODE_i input uint8; ATR_DURATION_i input uint16; ATR_FALLBACK_TIME_i input uint16; VENT_BLANKING_i input uint8; ACT_THRESHOLD_i input uint8; REACTION_TIME_i input uint8; RESPONSE_FACTOR_i input uint8; RECOVERY_TIME_i input uint16; PPARAM_UPDATE input boolean; ACTIVITY input double; STEP local double; B_LED output boolean; G_LED output boolean; R_LED output boolean; ACTIVITY_NORM local double; BPM local double; DIFF_MSR_LRL local double; MSR_ALTERED local double; VENT_PULSE_WIDTH local double; ATR_AMP_UNREG local double; ATR_DURATION local double; ATR_FALLBACK_TIME local double; ATR_MODE local double; AV_DELAY_DYNAMIC local double; AV_DELAY_FIXED local double; AV_DELAY_OFFSET_SENSED local double; HYSTERESIS_LIMIT local double; MIN_AV_DELAY_DYNAMIC local double; PVARP_EXT local double; PVARP local double; VENT_BLANKING local double; RATE_SMOOTHING local double; VENT_AMP_UNREG local double; VENT_SENSITIVITY local double; VRP local double; ACT_THRESHOLD local double; ARP local double; ATR_AMP_REG local double; ATR_PULSE_WIDTH local double; ATR_SENSITIVITY local double; LRL local double; MAX_SENSOR_RATE local double; REACTION_TIME local double; RECOVERY_TIME local double; RESPONSE_FACTOR local double; URL local double; VENT_AMP_REG local double; TARGET_HIGH local double; TARGET_LOW local double; SLOPE_DOWN local double; SLOPE_UP local double; ACT_V_HIGH constant double size=1 =2; ACT_HIGH constant double size=1 =1.75; ACT_M_HIGH constant double size=1 =1.5; ACT_M constant double size=1 =1.25; ACT_LOW constant double size=1 =1.2; ACT_M_LOW constant double size=1 =1.1; ACT_V_LOW constant double size=1 =1.05
